simulink library "bdotController_lib"  (R2018b)
settings: Solver=ode45  StartTime=0.0  StopTime=10.0  RelTol=1e-3  EnableMultiTasking=on
undefined symbols (not defined in the file or in its folder): fswParams
libraries: simulink x1
settings Model: Creator=Taylor  LastModifiedBy=taylorreynolds
settings DataIOCC: LimitDataPoints=on
settings OptimizationCC: LifeSpan=inf
settings DebuggingCC: AllowSymbolicDim=off  SFUnexpectedBacktrackingDiag=warning  SFNoUnconditionalDefaultTransitionDiag=warning  SFExecutionAtInitializationDiag=none
settings SFSimCC: SimUseLocalCustomCode=off
settings RTWCC: RTWUseLocalCustomCode=off
settings CodeAppCC: StateflowObjectComments=on
settings GRTTargetCC: TargetLangStandard=C89/C90 (ANSI)  GeneratePreprocessorConditionals=Disable all
settings ConfigComp: CovMetricSettings=dw  CovHtmlReporting=on  CovSaveCumulativeToWorkspaceVar=on  CovSaveSingleToWorkspaceVar=on  CovExternalEMLEnable=off

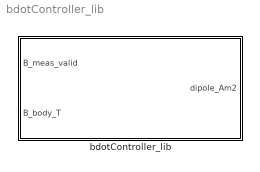
== system bdotController_lib ==
  bdotController_lib : Subsystem

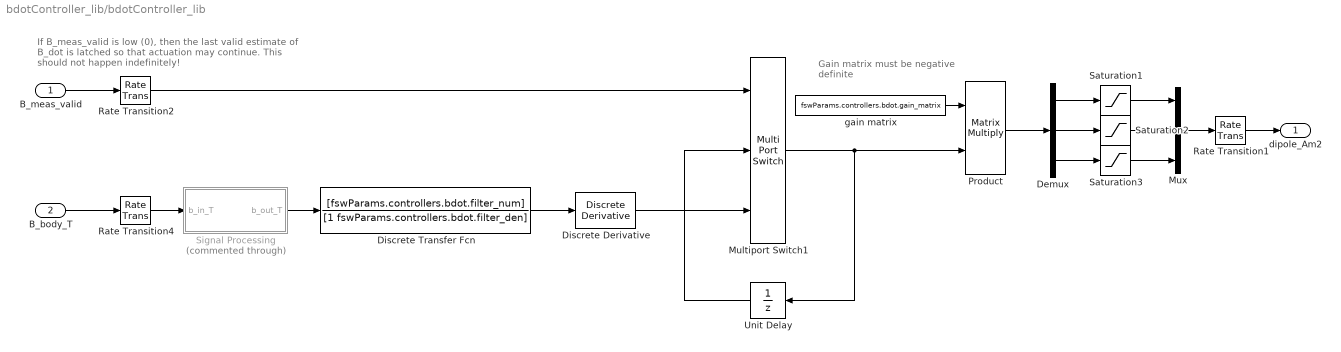
== system bdotController_lib/bdotController_lib ==
  note: If B_meas_valid is low (0), then the last valid
      | estimate of B_dot is latched so that actuation
      | may continue. This should not happen indefinitely!
  note: Gain matrix must be
      | negative definite
  B_meas_valid : Inport
  B_body_T : Inport  Port=2
  Demux : Demux  Outputs=3
  Discrete Transfer Fcn : DiscreteTransferFcn  Numerator=[fswParams.controllers.bdot.filter_num]  Denominator=[1 fswParams.controllers.bdot.filter_den]
  Discrete Derivative : simulink/Discrete/Discrete Derivative  gainval=1.0  ICPrevScaledInput=fswParams.controllers.bdot.ic.derivative  OutMin=[]  OutMax=[]  OutDataType=fixdt(1, 16)  OutScaling=2^-10  DoSatur=off
  Multiport Switch1 : MultiPortSwitch  DataPortOrder=Zero-based contiguous  Inputs=2  zeroidx=on
  Mux : Mux  Inputs=3
  Product : Product  Multiplication=Matrix(*)
  Rate Transition1 : RateTransition  InitialCondition=fswParams.controllers.bdot.ic.RT_dipole  OutPortSampleTimeOpt=Inherit  OutPortSampleTime=sc_params.control.sample_time_s
  Rate Transition2 : RateTransition  Deterministic=off  InitialCondition=fswParams.controllers.bdot.ic.RT_b_meas_valid  OutPortSampleTime=fswParams.controllers.bdot.sample_time_s
  Rate Transition4 : RateTransition  Deterministic=off  InitialCondition=fswParams.controllers.bdot.ic.RT_b_body_T  OutPortSampleTime=fswParams.controllers.bdot.sample_time_s
  Saturation1 : Saturate  UpperLimit=fswParams.actuators.mtq.max_dipole_x  LowerLimit=-fswParams.actuators.mtq.max_dipole_x
  Saturation2 : Saturate  UpperLimit=fswParams.actuators.mtq.max_dipole_y  LowerLimit=-fswParams.actuators.mtq.max_dipole_y
  Saturation3 : Saturate  UpperLimit=fswParams.actuators.mtq.max_dipole_z  LowerLimit=-fswParams.actuators.mtq.max_dipole_z
  Signal Processing : Subsystem  Commented=through
  Unit Delay : UnitDelay  InitialCondition=fswParams.controllers.bdot.ic.unit_delay  SampleTime=-1
  gain matrix : Constant  Value=fswParams.controllers.bdot.gain_matrix
  dipole_Am2 : Outport
  wires:
  Saturation1/1 -> Mux/1
  Unit Delay/1 -> Multiport Switch1/2
  Rate Transition1/1 -> dipole_Am2/1
  Rate Transition4/1 -> Signal Processing/1(b_in_T)
  B_body_T/1 -> Rate Transition4/1
  B_meas_valid/1 -> Rate Transition2/1
  Discrete Transfer Fcn/1 -> Discrete Derivative/1
  Discrete Derivative/1 -> Multiport Switch1/3
  Signal Processing/1(b_out_T) -> Discrete Transfer Fcn/1
  Multiport Switch1/1 -> Product/2, Unit Delay/1
  gain matrix/1 -> Product/1
  Product/1 -> Demux/1
  Demux/1 -> Saturation1/1
  Demux/3 -> Saturation3/1
  Demux/2 -> Saturation2/1
  Saturation3/1 -> Mux/3
  Saturation2/1 -> Mux/2
  Mux/1 -> Rate Transition1/1
  Rate Transition2/1 -> Multiport Switch1/1

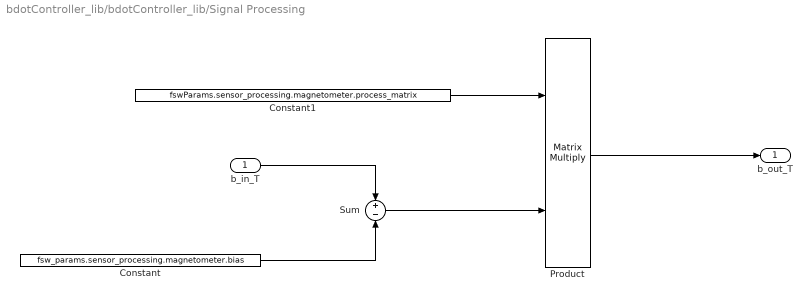
== system bdotController_lib/bdotController_lib/Signal Processing ==
  b_in_T : Inport
  Constant : Constant  Value=fsw_params.sensor_processing.magnetometer.bias  SampleTime=fswParams.controllers.bdot.sample_time_s
  Constant1 : Constant  Value=fswParams.sensor_processing.magnetometer.process_matrix  SampleTime=fswParams.controllers.bdot.sample_time_s
  Product : Product  Multiplication=Matrix(*)
  Sum : Sum  Inputs=+-
  b_out_T : Outport
  wires:
  Constant/1 -> Sum/2
  b_in_T/1 -> Sum/1
  Constant1/1 -> Product/1
  Sum/1 -> Product/2
  Product/1 -> b_out_T/1
